simulink model "Alineal_control_automatico"  (R2018a)
settings: Solver=VariableStepAuto  StartTime=0.0  StopTime=100  RelTol=1e-3
values from neighbouring files (symbols this model uses):
  g = 10    [derivador.m]
  L = 1    [derivador.m]    (also in ej_parcial.m = PC)
  m = 0.2    [derivador.m]
  R = 4    [derivador.m]
undefined symbols (not defined in the file or in its folder): magnitude
settings Model: Creator=Usuario  LastModifiedBy=Usuario

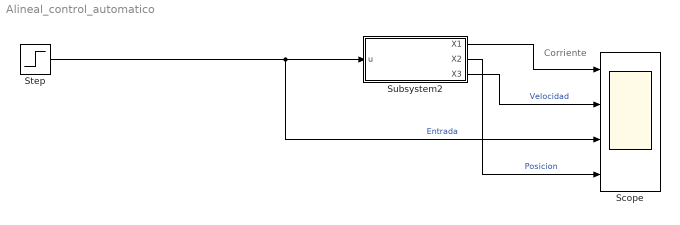
== system Alineal_control_automatico ==
  note: Corriente
  Scope : Scope  NumInputPorts=4
  Step : Step  Time=0  SampleTime=0
  Subsystem2 : Subsystem
  wires:
  Step/1 -> Scope/3, Subsystem2/1(u)  "Entrada"
  Subsystem2/1(X1) -> Scope/1
  Subsystem2/2("X2 ") -> Scope/4  "Posicion"
  Subsystem2/3("X3 ") -> Scope/2  "Velocidad"

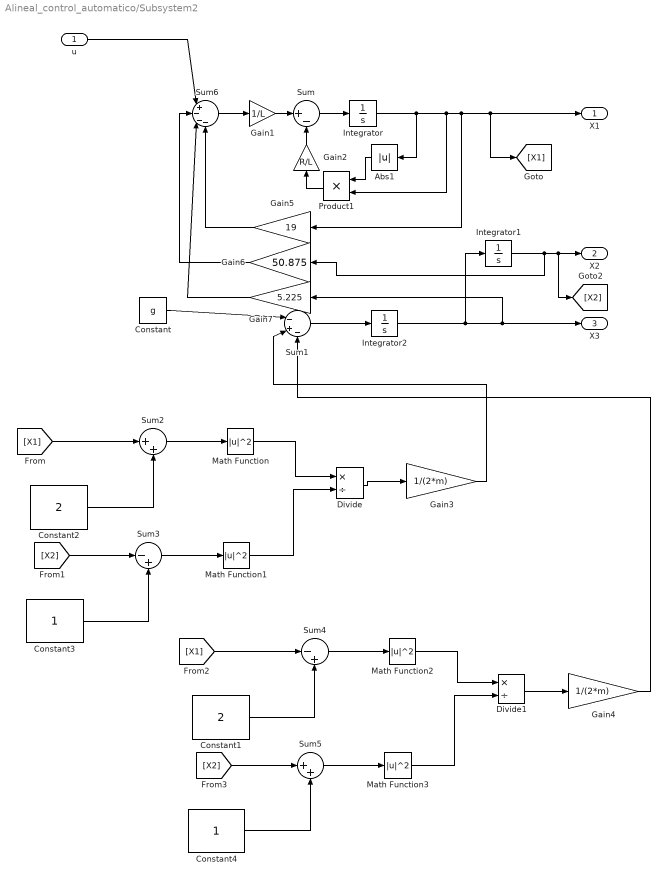
== system Alineal_control_automatico/Subsystem2 ==
  u : Inport
  Abs1 : Abs
  Constant : Constant  Value=g
  Constant1 : Constant  Value=2
  Constant2 : Constant  Value=2
  Constant3 : Constant
  Constant4 : Constant
  Divide : Product  Inputs=*/  SaturateOnIntegerOverflow=on  RndMeth=Zero
  Divide1 : Product  Inputs=*/  SaturateOnIntegerOverflow=on  RndMeth=Zero
  Gain1 : Gain  Gain=1/L
  Gain2 : Gain  Gain=R/L
  Gain3 : Gain  Gain=1/(2*m)
  Gain4 : Gain  Gain=1/(2*m)
  Gain5 : Gain  Gain=19
  Gain6 : Gain  Gain=50.875
  Gain7 : Gain  Gain=5.225
  Integrator : Integrator  InitialCondition=0.5
  Integrator1 : Integrator
  Integrator2 : Integrator
  Math Function{,1..3} (4 alike) : Math  Operator=magnitude^2  RndMeth=Zero  SaturateOnIntegerOverflow=on
  Product1 : Product
  Sum : Sum  Inputs=|+-
  Sum1 : Sum  Inputs=|-+-
  Sum2 : Sum  Inputs=|++
  Sum3 : Sum  Inputs=|-+
  Sum4 : Sum  Inputs=|-+
  Sum5 : Sum  Inputs=|++
  Sum6 : Sum  Inputs=|+---
  X1 : Outport
  "X2 " : Outport  Port=2
  "X3 " : Outport  Port=3
  wires:
  Gain1/1 -> Sum/1
  Sum/1 -> Integrator/1
  Abs1/1 -> Product1/1
  Integrator/1 -> Gain5/1, [X1], X1/1, Product1/2, Abs1/1
  Product1/1 -> Gain2/1
  Gain2/1 -> Sum/2
  Integrator1/1 -> Gain6/1, [X2], "X2 "/1
  Constant/1 -> Sum1/1
  [X1] -> Sum2/1
  Constant2/1 -> Sum2/2
  Sum2/1 -> Math Function/1
  [X2] -> Sum3/1
  Constant3/1 -> Sum3/2
  Sum3/1 -> Math Function1/1
  Sum1/1 -> Integrator2/1
  Math Function/1 -> Divide/1
  Math Function1/1 -> Divide/2
  Divide/1 -> Gain3/1
  Gain3/1 -> Sum1/2
  [X2] -> Sum5/1
  Sum4/1 -> Math Function2/1
  Math Function3/1 -> Divide1/2
  Sum5/1 -> Math Function3/1
  Math Function2/1 -> Divide1/1
  [X1] -> Sum4/1
  Constant4/1 -> Sum5/2
  Divide1/1 -> Gain4/1
  Constant1/1 -> Sum4/2
  Gain4/1 -> Sum1/3
  Integrator2/1 -> Gain7/1, "X3 "/1, Integrator1/1
  u/1 -> Sum6/1
  Sum6/1 -> Gain1/1
  Gain5/1 -> Sum6/4
  Gain6/1 -> Sum6/2
  Gain7/1 -> Sum6/3
